simulink model "ME322_Exercise_3_Stall_Case_Simulink"  (R2024b)
settings: Solver=VariableStepAuto  StartTime=0.0  StopTime=0.025  RelTol=1e-3
undefined symbols (not defined in the file or in its folder): u_stall, x_stall
settings Model: Creator=caidenbonney  LastModifiedBy=Caide

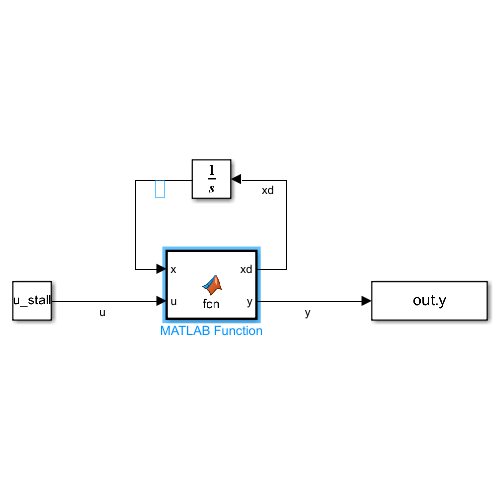
[thumbnail: Simulink's stored preview of the top-level diagram]
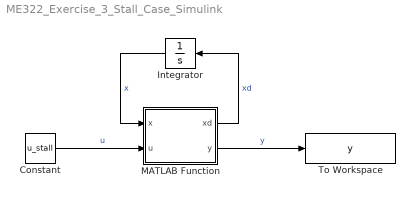
== system ME322_Exercise_3_Stall_Case_Simulink ==
  Constant : Constant  Value=u_stall  VectorParams1D=off
  Integrator : Integrator  InitialCondition=x_stall
  MATLAB Function : MATLAB Function  TreatAsAtomicUnit=on
  To Workspace : ToWorkspace  VariableName=y  SampleTime=-1
  wires:
  Constant/1 -> MATLAB Function/2(u)  "u"
  MATLAB Function/1(xd) -> Integrator/1  "xd"
  Integrator/1 -> MATLAB Function/1(x)  "x"
  MATLAB Function/2(y) -> To Workspace/1  "y"

== matlab function ME322_Exercise_3_Stall_Case_Simulink/MATLAB Function ==
  data: x input; xd output size=1; u input; y output size=5; p parameter
function [xd, y]= fcn(x, u, p)

% Separate state variables into individual elements
i_L = x(1);  % [A]
omega_J = 0; % [rad/sec]

% Separate input variables into individual elements
v_m = u(1); % [V]
T_L = 0;    % [N*m]

% Required given constants units
% p.L_m % [mH]
L_m = p.L_m *10^-3;  % [mH] -> 10^-3 [H]
% p.R_m % [ohms]

% State Equations
id_L = (1/(L_m))*(v_m - p.R_m*i_L); % <-- State eq. f_1
    % the expected units of the derivative of current with respect to
    % time is [A/sec]
        % (1/[H])    *    ([V] - [ohms]*[A])
        % (1/[V/(A/sec)])*([V] -  [V/A]*[A])
        % ([(A/sec)/V]  * ([V] - [V])
        % ([(A/sec)/V)*[V]
        % [A/sec]

xd = [id_L];      % <-- State f_1 [A/sec]

% Output Equations
P_e = v_m*i_L;        % <-- Output eq. g_3 Unit Check [V]*[A] = [W]
P_L = T_L*omega_J;    % <-- Output eq. g_4 Unit Check [N*m]*[rad/sec] = [W]
efficiency = P_L/P_e; % <-- Output eq. g_5 Unit Check [w]/[W] = [-]

y = [i_L          % <-- Output g_1 [A]
     omega_J      % <-- Output g_2 [rad/sec]
     P_e          % <-- Output g_3 [W]
     P_L          % <-- Output g_4 [W]
     efficiency]; % <-- Output g_5 [-]
